simulink model "cocosimLibs"  (R2015a)
settings: Solver=ode45  StartTime=0.0  StopTime=10.0  RelTol=1e-3
settings Model: Creator=Teme  LastModifiedBy=hbourbou
settings RTWCC: Toolchain=Clang v3.1 | gmake (64-bit Mac)

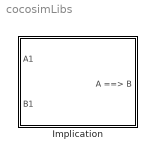
== system cocosimLibs ==
  Implication : Subsystem  mask(CoCoSim-Implies){}
      mask help: CoCoSim block for Logical Implication
      mask Display: disp(' ')

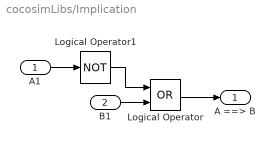
== system cocosimLibs/Implication ==
  A1 : Inport
  B1 : Inport  Port=2
  Logical Operator : Logic  Operator=OR  AllPortsSameDT=off  OutDataTypeStr=boolean
  Logical Operator1 : Logic  Operator=NOT  AllPortsSameDT=off  OutDataTypeStr=boolean
  A ==> B : Outport
  wires:
  A1/1 -> Logical Operator1/1
  Logical Operator1/1 -> Logical Operator/1
  B1/1 -> Logical Operator/2
  Logical Operator/1 -> A ==> B/1
